simulink library "pmm"  (R2021b)
settings: Solver=VariableStepAuto  StartTime=0.0  StopTime=10.0  RelTol=1e-3
undefined symbols (not defined in the file or in its folder): ENUM_ACMAINRLYSTS_OPEN, ENUM_ACPRECHRGRLYSTS_OPEN, ENUM_B2VRLYSTA_OPEN, ENUM_BMSHVSTS_HVOPEN, ENUM_BRAKEPEDAL_RELEASED, ENUM_CACRLYDEM_CLOSE, ENUM_CACRLYSTS_OPEN, ENUM_CHRGFAULT_ACRLYFAIL, ENUM_CHRGFAULT_BCUHVFAIL, ENUM_CHRGFAULT_BCUNEGFAIL, ENUM_CHRGFAULT_BCUTIMEOUT, ENUM_CHRGFAULT_DCDCENABLE, ENUM_CHRGFAULT_DCDCRLYFAIL, ENUM_CHRGFAULT_HVILFAIL, ENUM_CHRGFAULT_PDUHVFAIL, ENUM_CHRGFAULT_RLYCHKFAIL, ENUM_DCDCEACPCURLYSTA_CLOSED, ENUM_DCDCEACPCURLYSTA_FAILTOCLOSE, ENUM_DCDCEACPCURLYSTA_OPEN, ENUM_DCDCEACPCURLYSTA_WELDED, ENUM_DCDCENABLESTS_READY, ENUM_DCDCRLYSTS_OPEN, ENUM_EHPSRLYDEM_CLOSE, ENUM_EHPSRLYSTS_OPEN, ENUM_FOGRLYENCMD_DISABLE, ENUM_GEARACTUALPOSN_D, ENUM_HVPWROFFREQ_POWEROFF, ENUM_KEYSTATUS_OFF, ENUM_KEYSTATUS_ON, ENUM_KEYSTATUS_START, ENUM_LOWBATTVOLTAGE_NORMAL, ENUM_LOWBATTVOLTAGE_POWERDOWN, ENUM_LOWBATTVOLTAGE_POWERUP, ENUM_MCUHVLOOP_POWEROFF, ENUM_MCUHVLOOPSTS_OPEN, ENUM_MCUMAINRLYSTS_OPEN, ENUM_MCUPRECHRGRLYSTS_OPEN, ENUM_PDFAULT_ACRLYOPEN, ENUM_PDFAULT_BCUDISABLE, ENUM_PDFAULT_DCDCDISABLE, ENUM_PDFAULT_DCDCRLYOPEN, ENUM_PDFAULT_EACDISABLE, ENUM_PDFAULT_EACRLYOPEN, ENUM_PDFAULT_EHPSDISABLE, ENUM_PDFAULT_EHPSRLYOPEN, ENUM_PDFAULT_MCUDISABLE, ENUM_PDFAULT_MCUDISCHRG, ENUM_PDFAULT_MCURLYOPEN, ENUM_PEUSELFCHKSTS_NOFAULT, ENUM_PLUGINSTS_NOPLUGIN, ENUM_PLUGINSTS_PLUGIN, ENUM_PMMMODE_DRIVE, ENUM_PMMMODE_LVBATCHRG, ENUM_PUSTATE_DCDCENABLE, ENUM_PUSTATE_EACPRESCHECK, ENUM_PUSTATE_EHPSENABLE, ENUM_PUSTATE_MCUENABLE, ENUM_PUSTATE_PDUMCURLYCLOSED, ENUM_PUSTATE_POWERUPFAIL, ENUM_TARGETGEAR_REVERSE ... (+126)
libraries: hcu_lib x45, simulink x5, ddm x1, dsc x1
(part 4 of 7)

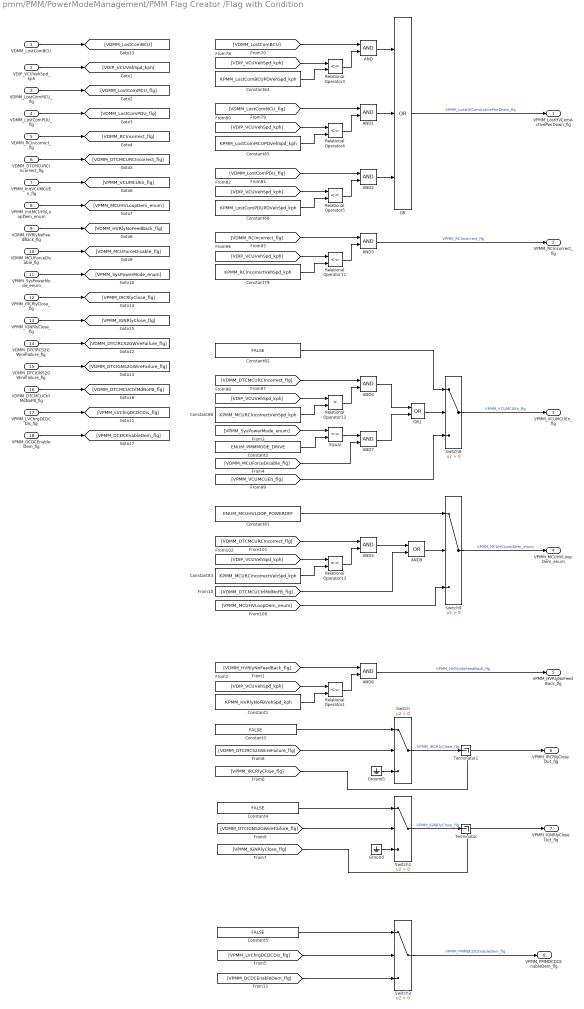
== system pmm/PMM/PowerModeManagement/PMM Flag Creator /Flag with Condition ==
  VDMM_LostComBCU : Inport
  VDIP_VCUVehSpd_kph : Inport  Port=2
  VDMM_LostComMCU_flg : Inport  Port=3
  VDMM_LostComPDU_flg : Inport  Port=4
  VDMM_RCIncorrect_flg : Inport  Port=5
  VDMM_DTCMCURCIncorrect_flg : Inport  Port=6
  VPMM_InitVCUMCUEn_flg : Inport  Port=7
  VPMM_InitMCUHVLoopDem_enum : Inport  Port=8
  VDMM_HVRlyNoFeedBack_flg : Inport  Port=9
  VDMM_MCUForceDisable_flg : Inport  Port=10
  VPMM_SysPowerMode_enum : Inport  Port=11
  VPMM_IRCRlyClose_flg : Inport  Port=12
  VPMM_IGNRlyClose_flg : Inport  Port=13
  VDMM_DTCIRCS2GWireFailure_flg : Inport  Port=14
  VDMM_DTCIGNS2GWireFailure_flg : Inport  Port=15
  VDMM_DTCMCUCtrlMdNoFB_flg : Inport  Port=16
  VPMM_LVChrgDCDCDis_flg : Inport  Port=17
  VPMM_DCDCEnableDem_flg : Inport  Port=18
  AND{,1..7} (8 alike) : Logic  AllPortsSameDT=off  OutDataTypeStr=boolean
  AND9 : Logic  Operator=OR  AllPortsSameDT=off  OutDataTypeStr=boolean
  Constant1 : Constant  Value=KPMM_HVRlyNoFBVehSpd_kph
  Constant2 : Constant  Value=ENUM_PMMMODE_DRIVE
  Constant{3..5,82} (4 alike) : Constant  Value=FALSE
  Constant64 : Constant  Value=KPMM_LostComBCUPDVehSpd_kph
  Constant65 : Constant  Value=KPMM_LostComMCUPDVehSpd_kph
  Constant66 : Constant  Value=KPMM_LostComPDUPDVehSpd_kph
  Constant79 : Constant  Value=KPMM_RCIncorrectVehSpd_kph
  Constant80 : Constant  Value=KPMM_MCURCIncorrectVehSpd_kph
  Constant81 : Constant  Value=ENUM_MCUHVLOOP_POWEROFF
  Constant83 : Constant  Value=KPMM_MCURCIncorrectVehSpd_kph
  Equal : RelationalOperator  Operator===  OutDataTypeStr=boolean  RndMeth=Simplest
  Ground : Ground
  Ground1 : Ground
  OR : Logic  Operator=OR  Inputs=3  AllPortsSameDT=off  OutDataTypeStr=boolean
  OR1 : Logic  Operator=OR  AllPortsSameDT=off  OutDataTypeStr=boolean
  Relational Operator{1,3..5,11,13} (6 alike) : RelationalOperator  Operator=<=  OutDataTypeStr=boolean  RndMeth=Simplest
  Relational Operator12 : RelationalOperator  Operator=>  OutDataTypeStr=boolean  RndMeth=Simplest
  Switch{,1..2,8..9} (5 alike) : Switch  Criteria=u2 > Threshold
  Terminator : Terminator
  Terminator1 : Terminator
  VPMM_LostHVComActivePwrDown_flg : Outport
  VPMM_RCIncorrect_flg : Outport  Port=2
  VPMM_VCUMCUEn_flg : Outport  Port=3
  VPMM_MCUHVLoopDem_enum : Outport  Port=4
  VPMM_HVRlyNoFeedBack_flg : Outport  Port=5
  VPMM_IRCRlyCloseOut_flg : Outport  Port=6
  VPMM_IGNRlyCloseOut_flg : Outport  Port=7
  VPMM_PMMDCDCEnableDem_flg : Outport  Port=8
  wires:
  Relational Operator11/1 -> AND3/2
  Relational Operator4/1 -> AND1/2
  Constant79/1 -> Relational Operator11/2
  AND/1 -> OR/1
  Relational Operator5/1 -> AND2/2
  [VDIP_VCUVehSpd_kph] -> Relational Operator3/1
  [VDIP_VCUVehSpd_kph] -> Relational Operator11/1
  Relational Operator12/1 -> AND4/2
  [VDMM_LostComPDU_flg] -> AND2/1
  [VDMM_DTCMCURCIncorrect_flg] -> AND5/1
  Constant65/1 -> Relational Operator4/2
  Constant83/1 -> Relational Operator13/2
  OR/1 -> VPMM_LostHVComActivePwrDown_flg/1  "VPMM_LostHVComActivePwrDown_flg"
  [VDIP_VCUVehSpd_kph] -> Relational Operator12/1
  Constant80/1 -> Relational Operator12/2
  Relational Operator13/1 -> AND5/2
  Constant66/1 -> Relational Operator5/2
  [VDIP_VCUVehSpd_kph] -> Relational Operator5/1
  [VDMM_LostComBCU] -> AND/1
  Constant64/1 -> Relational Operator3/2
  AND2/1 -> OR/3
  Relational Operator3/1 -> AND/2
  [VDMM_LostComMCU_flg] -> AND1/1
  [VDMM_RCIncorrect_flg] -> AND3/1
  [VDIP_VCUVehSpd_kph] -> Relational Operator4/1
  [VDIP_VCUVehSpd_kph] -> Relational Operator13/1
  AND1/1 -> OR/2
  Switch8/1 -> VPMM_VCUMCUEn_flg/1  "VPMM_VCUMCUEn_flg"
  Switch9/1 -> VPMM_MCUHVLoopDem_enum/1  "VPMM_MCUHVLoopDem_enum"
  AND3/1 -> VPMM_RCIncorrect_flg/1  "VPMM_RCIncorrect_flg"
  VDMM_LostComBCU/1 -> [VDMM_LostComBCU]
  VDIP_VCUVehSpd_kph/1 -> [VDIP_VCUVehSpd_kph]
  VDMM_LostComMCU_flg/1 -> [VDMM_LostComMCU_flg]
  VDMM_LostComPDU_flg/1 -> [VDMM_LostComPDU_flg]
  VDMM_RCIncorrect_flg/1 -> [VDMM_RCIncorrect_flg]
  VDMM_DTCMCURCIncorrect_flg/1 -> [VDMM_DTCMCURCIncorrect_flg]
  VPMM_InitVCUMCUEn_flg/1 -> [VPMM_VCUMCUEn_flg]
  VPMM_InitMCUHVLoopDem_enum/1 -> [VPMM_MCUHVLoopDem_enum]
  AND6/1 -> VPMM_HVRlyNoFeedBack_flg/1  "VPMM_HVRlyNoFeedBack_flg"
  [VDMM_HVRlyNoFeedBack_flg] -> AND6/1
  [VDIP_VCUVehSpd_kph] -> Relational Operator1/1
  Constant1/1 -> Relational Operator1/2
  Relational Operator1/1 -> AND6/2
  VDMM_HVRlyNoFeedBack_flg/1 -> [VDMM_HVRlyNoFeedBack_flg]
  VDMM_MCUForceDisable_flg/1 -> [VDMM_MCUForceDisable_flg]
  VPMM_SysPowerMode_enum/1 -> [VPMM_SysPowerMode_enum]
  [VPMM_SysPowerMode_enum] -> Equal/1
  Constant2/1 -> Equal/2
  Equal/1 -> AND7/1
  [VDMM_MCUForceDisable_flg] -> AND7/2
  OR1/1 -> Switch8/2
  AND4/1 -> OR1/1
  AND7/1 -> OR1/2
  [VPMM_VCUMCUEn_flg] -> Switch8/3
  Constant82/1 -> Switch8/1
  [VDMM_DTCMCURCIncorrect_flg] -> AND4/1
  VDMM_DTCIGNS2GWireFailure_flg/1 -> [VDMM_DTCIGNS2GWireFailure_flg]
  VDMM_DTCIRCS2GWireFailure_flg/1 -> [VDMM_DTCIRCS2GWireFailure_flg]
  VPMM_IGNRlyClose_flg/1 -> [VPMM_IGNRlyClose_flg]
  VPMM_IRCRlyClose_flg/1 -> [VPMM_IRCRlyClose_flg]
  [VDMM_DTCIRCS2GWireFailure_flg] -> Switch/2
  Constant3/1 -> Switch/1
  Constant4/1 -> Switch1/1
  VDMM_DTCMCUCtrlMdNoFB_flg/1 -> [VDMM_DTCMCUCtrlMdNoFB_flg]
  AND5/1 -> AND9/1
  AND9/1 -> Switch9/2
  [VDMM_DTCMCUCtrlMdNoFB_flg] -> AND9/2
  [VPMM_MCUHVLoopDem_enum] -> Switch9/3
  Constant81/1 -> Switch9/1
  [VDMM_DTCIGNS2GWireFailure_flg] -> Switch1/2
  [VPMM_IGNRlyClose_flg] -> VPMM_IGNRlyCloseOut_flg/1
  Switch1/1 -> Terminator/1  "VPMM_IGNRlyClose_flg"
  Ground/1 -> Switch1/3
  [VPMM_IRCRlyClose_flg] -> VPMM_IRCRlyCloseOut_flg/1
  Ground1/1 -> Switch/3
  Switch/1 -> Terminator1/1  "VPMM_IRCRlyClose_flg"
  VPMM_LVChrgDCDCDis_flg/1 -> [VPMM_LVChrgDCDCDis_flg]
  [VPMM_LVChrgDCDCDis_flg] -> Switch2/2
  Constant5/1 -> Switch2/1
  VPMM_DCDCEnableDem_flg/1 -> [VPMM_DCDCEnableDem_flg]
  [VPMM_DCDCEnableDem_flg] -> Switch2/3
  Switch2/1 -> VPMM_PMMDCDCEnableDem_flg/1  "VPMM_PMMDCDCEnableDem_flg"

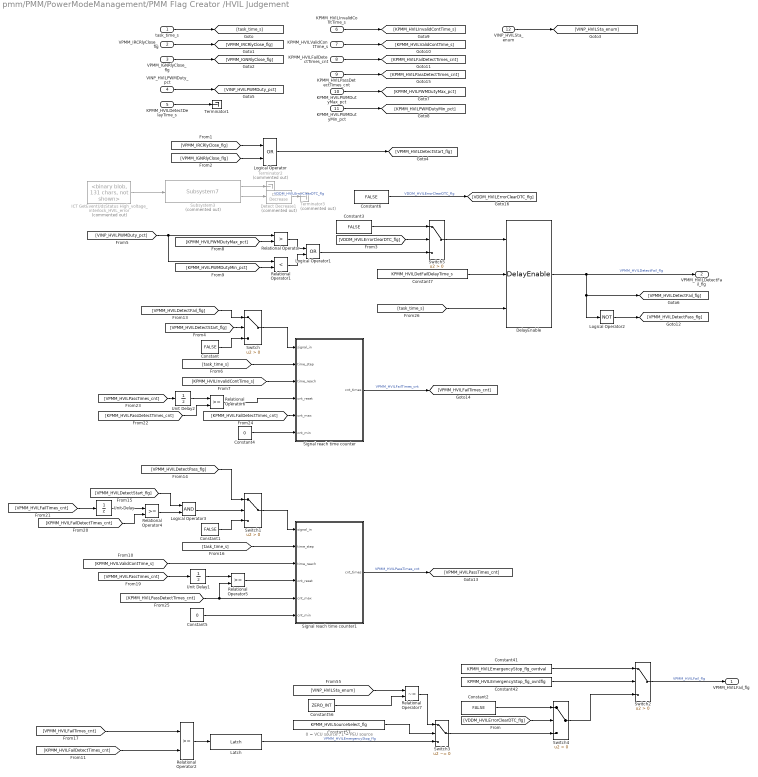
== system pmm/PMM/PowerModeManagement/PMM Flag Creator /HVIL Judgement ==
  note: 0 = VCU source；1 = PEU source
  task_time_s : Inport
  VPMM_IRCRlyClose_flg : Inport  Port=2
  VPMM_IGNRlyClose_flg : Inport  Port=3
  VINP_HVILPWMDuty_pct : Inport  Port=4
  KPMM_HVILDetectDelayTime_s : Inport  Port=5
  KPMM_HVILInvalidContTime_s : Inport  Port=6
  KPMM_HVILValidContTime_s : Inport  Port=7
  KPMM_HVILFailDetectTimes_cnt : Inport  Port=8
  KPMM_HVILPassDetectTimes_cnt : Inport  Port=9
  KPMM_HVILPWMDutyMax_pct : Inport  Port=10
  KPMM_HVILPWMDutyMin_pct : Inport  Port=11
  VINP_HVILSta_enum : Inport  Port=12
  Constant{,1..3,6} (5 alike) : Constant  Value=FALSE
  Constant4 : Constant  Value=0  OutDataTypeStr=single
  Constant41 : Constant  Value=KPMM_HVILEmergencyStop_flg_ovrdval
  Constant42 : Constant  Value=KPMM_HVILEmergencyStop_flg_ovrdflg
  Constant5 : Constant  Value=0  OutDataTypeStr=single
  Constant56 : Constant  Value=ZERO_INT
  Constant57 : Constant  Value=KPMM_HVILSourceSelect_flg
  Constant7 : Constant  Value=KPMM_HVILDetFailDelayTime_s
  DelayEnable : hcu_lib/Basic_Blocks/DelayEnable
  Detect Decrease1 : simulink/Logic and Bit Operations/Detect Decrease  Commented=on  vinit=0.0  OutDataTypeStr=boolean
  ICT GetEventUdsStatus High_voltage_interlock_HVIL_error : ddm/DDM/DMM_Module/SOP3 Wire Failure Detection/Rolling Counting Error Clear/ICT GetEventUdsStatus High_voltage_interlock_HVIL_error  Commented=on  SystemSampleTime=-1  VariantActivationTime=update diagram  Latency=0  AutoFrameSizeCalculation=off
  Latch : hcu_lib/Basic_Blocks/Latch
  Logical Operator : Logic  Operator=OR  AllPortsSameDT=off  OutDataTypeStr=boolean
  Logical Operator1 : Logic  Operator=OR  AllPortsSameDT=off  OutDataTypeStr=boolean
  Logical Operator2 : Logic  Operator=NOT  AllPortsSameDT=off  OutDataTypeStr=boolean
  Logical Operator3 : Logic  AllPortsSameDT=off  OutDataTypeStr=boolean
  Relational Operator : RelationalOperator  Operator=>  OutDataTypeStr=boolean  RndMeth=Simplest
  Relational Operator1 : RelationalOperator  Operator=<  OutDataTypeStr=boolean  RndMeth=Simplest
  Relational Operator{2,4..6} (4 alike) : RelationalOperator  OutDataTypeStr=boolean  RndMeth=Simplest
  Relational Operator7 : RelationalOperator  Operator=~=  OutDataTypeStr=boolean  RndMeth=Simplest
  Signal reach time counter : Subsystem
  Signal reach time counter1 : Subsystem
  Subsystem3 : dsc/DSC/DSC/DTC_DMM/Subsystem7  Commented=on  SystemSampleTime=-1  VariantActivationTime=update diagram  Latency=0  AutoFrameSizeCalculation=off
  Switch{,1..2,4..5} (5 alike) : Switch  Criteria=u2 > Threshold
  Switch3 : Switch  Criteria=u2 ~= 0
      settings: AttributesFormatString=%<Criteria>
  Terminator1 : Terminator
  Terminator2 : Terminator  Commented=on
  Terminator3 : Terminator  Commented=on
  Unit Delay : UnitDelay  SampleTime=-1  HasFrameUpgradeWarning=on
  Unit Delay1 : UnitDelay  SampleTime=-1  HasFrameUpgradeWarning=on
  Unit Delay2 : UnitDelay  SampleTime=-1  HasFrameUpgradeWarning=on
  VPMM_HVILFail_flg : Outport
  VPMM_HVILDetectFail_flg : Outport  Port=2
  wires:
  Logical Operator1/1 -> Switch5/3
  [VDDM_HVILErrorClearDTC_flg] -> Switch5/2
  Constant3/1 -> Switch5/1
  Switch4/1 -> Switch2/3
  Constant2/1 -> Switch4/1
  [VDDM_HVILErrorClearDTC_flg] -> Switch4/2
  Switch3/1 -> Switch4/3
  Constant6/1 -> [VDDM_HVILErrorClearDTC_flg]  "VDDM_HVILErrorClearDTC_flg"
  Subsystem3/2 -> Detect Decrease1/1
  ICT GetEventUdsStatus High_voltage_interlock_HVIL_error/1 -> Subsystem3/1
  Subsystem3/1 -> Terminator2/1
  Unit Delay2/1 -> Relational Operator6/1
  Unit Delay1/1 -> Relational Operator5/1
  Unit Delay/1 -> Relational Operator4/1
  [VPMM_HVILPassTimes_cnt] -> Unit Delay2/1
  [KPMM_HVILPassDetectTimes_cnt] -> Relational Operator6/2
  Relational Operator6/1 -> Signal reach time counter/4(cnt_reset)
  [VPMM_HVILPassTimes_cnt] -> Unit Delay1/1
  Logical Operator3/1 -> Switch1/2
  [VPMM_HVILDetectStart_flg] -> Logical Operator3/1
  [KPMM_HVILFailDetectTimes_cnt] -> Relational Operator4/2
  Relational Operator4/1 -> Logical Operator3/2
  [VPMM_HVILFailTimes_cnt] -> Unit Delay/1
  Relational Operator5/1 -> Signal reach time counter1/4(cnt_reset)
  Relational Operator2/1 -> Latch/1
  [KPMM_HVILFailDetectTimes_cnt] -> Relational Operator2/2
  [VPMM_HVILFailTimes_cnt] -> Relational Operator2/1
  KPMM_HVILPassDetectTimes_cnt/1 -> [KPMM_HVILPassDetectTimes_cnt]
  [KPMM_HVILValidContTime_s] -> Signal reach time counter1/3(time_reach)
  [task_time_s] -> Signal reach time counter1/2(time_step)
  [VPMM_HVILDetectPass_flg] -> Switch1/1
  Switch1/1 -> Signal reach time counter1/1(signal_in)
  Constant1/1 -> Switch1/3
  [KPMM_HVILPassDetectTimes_cnt] -> Signal reach time counter1/5(cnt_max), Relational Operator5/2
  Constant5/1 -> Signal reach time counter1/6(cnt_min)
  Signal reach time counter1/1(cnt_times) -> [VPMM_HVILPassTimes_cnt]  "VPMM_HVILPassTimes_cnt"
  Signal reach time counter/1(cnt_times) -> [VPMM_HVILFailTimes_cnt]  "VPMM_HVILFailTimes_cnt"
  Constant4/1 -> Signal reach time counter/6(cnt_min)
  [KPMM_HVILFailDetectTimes_cnt] -> Signal reach time counter/5(cnt_max)
  Constant/1 -> Switch/3
  [VPMM_HVILDetectStart_flg] -> Switch/2
  Switch/1 -> Signal reach time counter/1(signal_in)
  [VPMM_HVILDetectFail_flg] -> Switch/1
  [task_time_s] -> Signal reach time counter/2(time_step)
  [KPMM_HVILInvalidContTime_s] -> Signal reach time counter/3(time_reach)
  Logical Operator2/1 -> [VPMM_HVILDetectPass_flg]
  Relational Operator1/1 -> Logical Operator1/2
  Relational Operator/1 -> Logical Operator1/1
  [KPMM_HVILPWMDutyMin_pct] -> Relational Operator1/2
  [KPMM_HVILPWMDutyMax_pct] -> Relational Operator/2
  [VINP_HVILPWMDuty_pct] -> Relational Operator/1, Relational Operator1/1
  KPMM_HVILFailDetectTimes_cnt/1 -> [KPMM_HVILFailDetectTimes_cnt]
  KPMM_HVILValidContTime_s/1 -> [KPMM_HVILValidContTime_s]
  KPMM_HVILInvalidContTime_s/1 -> [KPMM_HVILInvalidContTime_s]
  KPMM_HVILPWMDutyMin_pct/1 -> [KPMM_HVILPWMDutyMin_pct]
  KPMM_HVILPWMDutyMax_pct/1 -> [KPMM_HVILPWMDutyMax_pct]
  VINP_HVILPWMDuty_pct/1 -> [VINP_HVILPWMDuty_pct]
  Logical Operator/1 -> [VPMM_HVILDetectStart_flg]
  KPMM_HVILDetectDelayTime_s/1 -> Terminator1/1
  [VPMM_IGNRlyClose_flg] -> Logical Operator/2
  [VPMM_IRCRlyClose_flg] -> Logical Operator/1
  VPMM_IGNRlyClose_flg/1 -> [VPMM_IGNRlyClose_flg]
  VPMM_IRCRlyClose_flg/1 -> [VPMM_IRCRlyClose_flg]
  task_time_s/1 -> [task_time_s]
  Relational Operator7/1 -> Switch3/1
  [VINP_HVILSta_enum] -> Relational Operator7/1
  Switch2/1 -> VPMM_HVILFail_flg/1  "VPMM_HVILFail_flg"
  Constant57/1 -> Switch3/2
  Constant56/1 -> Relational Operator7/2
  Constant41/1 -> Switch2/1
  Latch/1 -> Switch3/3  "VPMM_HVILEmergencyStop_flg"
  Constant42/1 -> Switch2/2
  VINP_HVILSta_enum/1 -> [VINP_HVILSta_enum]
  Detect Decrease1/1 -> Terminator3/1  "VDDM_HVILErrorClearDTC_flg"
  Switch5/1 -> DelayEnable/1
  DelayEnable/1 -> Logical Operator2/1, [VPMM_HVILDetectFail_flg], VPMM_HVILDetectFail_flg/1  "VPMM_HVILDetectFail_flg"
  [task_time_s] -> DelayEnable/3
  Constant7/1 -> DelayEnable/2

== system pmm/PMM/PowerModeManagement/PMM Flag Creator /Long Idle Detection ==
  VDIP_VCUVehSpd_kph : Inport
  VTQD_GearActualPosn_enum : Inport  Port=2
  VINP_EBSBrakeSw_enum : Inport  Port=3
  VINP_MotorSpd_rpm : Inport  Port=4
  VSCP_FRDoorOPSta_flg : Inport  Port=5
  VSCP_MDDoorOPSta_flg : Inport  Port=6
  VSCP_TDDoorOPSta_flg : Inport  Port=7
  VPMM_SysPowerMode_enum : Inport  Port=8
  task_time_s : Inport  Port=9
  AND : Logic  Inputs=4  AllPortsSameDT=off  OutDataTypeStr=boolean
  AND1 : Logic  Inputs=3  AllPortsSameDT=off  OutDataTypeStr=boolean
  AND2 : Logic  AllPortsSameDT=off  OutDataTypeStr=boolean
  Abs : Abs
  Constant : Constant  Value=KPMM_LongIdleDectVehSpd_kph
  Constant1 : Constant  Value=ENUM_GEARACTUALPOSN_D
  Constant2 : Constant  Value=KPMM_LongIdleDectMotorSpd_rpm
  Constant3 : Constant  Value=ENUM_PMMMODE_DRIVE
  Constant4 : Constant  Value=KPMM_LongIdleDectTime_s
  Constant5 : Constant  Value=KPMM_LongIdleDetSW_flg
  Constant6 : Constant  Value=ENUM_BRAKEPEDAL_RELEASED
  Constant7 : Constant  Value=KPMM_LongIdleBuzzerFlashTime_s
  DelayEnable : hcu_lib/Basic_Blocks/DelayEnable
  DelayEnable1 : hcu_lib/Basic_Blocks/DelayEnable
  Equal : RelationalOperator  Operator===  OutDataTypeStr=boolean  RndMeth=Simplest
  Equal1 : RelationalOperator  Operator===  OutDataTypeStr=boolean  RndMeth=Simplest
  Equal2 : RelationalOperator  Operator===  OutDataTypeStr=boolean  RndMeth=Simplest
  Latch : hcu_lib/Basic_Blocks/Latch
  OR : Logic  Operator=OR  Inputs=3  AllPortsSameDT=off  OutDataTypeStr=boolean
  Relational Operator : RelationalOperator  Operator=<=  OutDataTypeStr=boolean  RndMeth=Simplest
  Relational Operator1 : RelationalOperator  Operator=<=  OutDataTypeStr=boolean  RndMeth=Simplest
  VPMM_LongIdleDetFinsh_flg : Outport
  VPMM_LongIdle_flg : Outport  Port=2
  wires:
  AND1/1 -> DelayEnable/1  "VPMM_LongIdleEn_flg"
  task_time_s/1 -> [task_time_s]
  [VDIP_VCUVehSpd_kph] -> Relational Operator/1
  [VPMM_LongIdleDoorCon_flg] -> AND1/2
  DelayEnable/1 -> Latch/1
  Latch/1 -> AND2/1
  Constant5/1 -> AND2/2
  Equal/1 -> AND/2
  Constant4/1 -> DelayEnable/2
  AND2/1 -> [VPMM_LongIdleDetFinsh_flg]  "VPMM_LongIdleDetFinsh_flg"
  OR/1 -> [VPMM_LongIdleDoorCon_flg]  "VPMM_LongIdleDoorCon_flg"
  VINP_EBSBrakeSw_enum/1 -> [VINP_EBSBrakeSw_enum]
  [VPMM_LongIdleDetFinsh_flg] -> VPMM_LongIdleDetFinsh_flg/1
  VDIP_VCUVehSpd_kph/1 -> [VDIP_VCUVehSpd_kph]
  Constant1/1 -> Equal/2
  Constant/1 -> Relational Operator/2
  Constant2/1 -> Relational Operator1/2
  VSCP_FRDoorOPSta_flg/1 -> [VSCP_FRDoorOPSta_flg]
  [VPMM_SysPowerMode_enum] -> Equal1/1
  VINP_MotorSpd_rpm/1 -> [VINP_MotorSpd_rpm]
  Abs/1 -> Relational Operator1/1
  Relational Operator1/1 -> AND/3
  Equal2/1 -> AND/4
  [VPMM_LongIdlePowerCon_flg] -> AND1/3
  Relational Operator/1 -> AND/1
  VSCP_MDDoorOPSta_flg/1 -> [VSCP_MDDoorOPSta_flg]
  Equal1/1 -> [VPMM_LongIdlePowerCon_flg]  "VPMM_LongIdlePowerCon_flg"
  AND/1 -> [VPMM_LongIdleDriveCon_flg]  "VPMM_LongIdleDriveCon_flg"
  VTQD_GearActualPosn_enum/1 -> [VTQD_GearActualPosn_enum]
  [VPMM_LongIdleDriveCon_flg] -> AND1/1
  VSCP_TDDoorOPSta_flg/1 -> [VSCP_TDDoorOPSta_flg]
  [task_time_s] -> DelayEnable/3
  VPMM_SysPowerMode_enum/1 -> [VPMM_SysPowerMode_enum]
  Constant3/1 -> Equal1/2
  Constant6/1 -> Equal2/2
  [VINP_MotorSpd_rpm] -> Abs/1
  [VINP_EBSBrakeSw_enum] -> Equal2/1
  [VTQD_GearActualPosn_enum] -> Equal/1
  [VPMM_LongIdleDetFinsh_flg] -> DelayEnable1/1
  Constant7/1 -> DelayEnable1/2
  [task_time_s] -> DelayEnable1/3
  DelayEnable1/1 -> [VPMM_LongIdle_flg]  "VPMM_LongIdle_flg"
  [VPMM_LongIdle_flg] -> VPMM_LongIdle_flg/1
  [VSCP_FRDoorOPSta_flg] -> OR/1
  [VSCP_MDDoorOPSta_flg] -> OR/2
  [VSCP_TDDoorOPSta_flg] -> OR/3

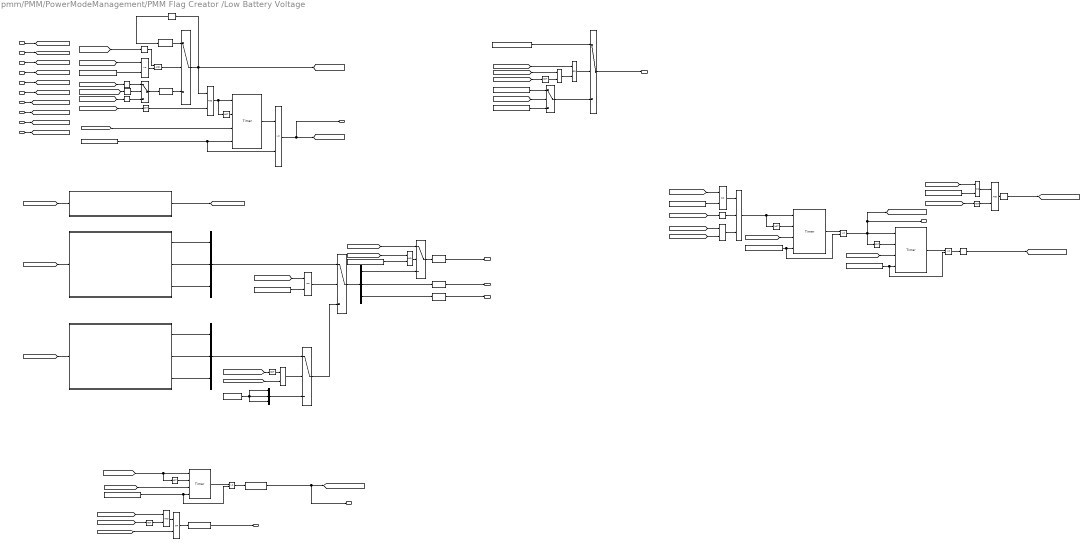
== system pmm/PMM/PowerModeManagement/PMM Flag Creator /Low Battery Voltage ==
  note: LVChrgMode Cycle Timer
  note: Battery Low Voltage Indicator
  note: Flasher
  note: Low Valtage Detection
  task_time_s : Inport
  VINP_DCDCOutVol_V : Inport  Port=2
  VINP_DCDCEnSta_enum : Inport  Port=3
  VPMM_LVChrgIinit2Idle_flg : Inport  Port=4
  VPMM_SysPowerMode_enum : Inport  Port=5
  VINP_B2VSOC_pct : Inport  Port=6
  VPMM_HVUnitSelfChkCompleted4PU_flg : Inport  Port=7
  VPMM_LVChrgInit2PowerUp_flg : Inport  Port=8
  VPMM_HVILFail_flg : Inport  Port=9
  VPMM_LongIdleDetFinsh_flg : Inport  Port=10
  AND{,1,4..8} (7 alike) : Logic  AllPortsSameDT=off  OutDataTypeStr=boolean
  AND2 : Logic  Inputs=3  AllPortsSameDT=off  OutDataTypeStr=boolean
  AND3 : Logic  Operator=NAND  AllPortsSameDT=off  OutDataTypeStr=boolean
  Constant1 : Constant  Value=ENUM_LOWBATTVOLTAGE_NORMAL  VectorParams1D=off
  Constant10 : Constant  Value=KPMM_LongIdleBuzzerSW_flg  VectorParams1D=off
  Constant2 : Constant  Value=ENUM_LOWBATTVOLTAGE_POWERUP  VectorParams1D=off
  Constant20 : Constant  Value=FALSE
  Constant3 : Constant  Value=KPMM_LVChrgPreAction_s  VectorParams1D=off
  Constant4 : Constant  Value=ENUM_LOWBATTVOLTAGE_POWERDOWN  VectorParams1D=off
  Constant5 : Constant  Value=ENUM_PMMMODE_LVBATCHRG  VectorParams1D=off
  Constant6 : Constant  Value=ENUM_PMMMODE_LVBATCHRG  VectorParams1D=off
  Constant7 : Constant  Value=KPMM_LVChrgDCDCEnTimer_s  VectorParams1D=off
  Constant76 : Constant  Value=KPMM_LVChrgPreAlarm_s  VectorParams1D=off
  Constant78 : Constant  Value=ENUM_DCDCENABLESTS_READY
  Constant8 : Constant  Value=KPMM_LVChrgDCDCDisTimer_s  VectorParams1D=off
  Constant9 : Constant  Value=ENUM_PMMMODE_LVBATCHRG  VectorParams1D=off
  Data Type Conversion{,1..4} (5 alike) : DataTypeConversion  OutDataTypeStr=boolean
  Delay{,1..4} (5 alike) : Delay  DelayLength=1
  Demux : Demux  Outputs=3
  Equal : RelationalOperator  Operator===  OutDataTypeStr=boolean  RndMeth=Simplest
  Equal1 : RelationalOperator  Operator===  OutDataTypeStr=boolean  RndMeth=Simplest
  Equal2 : RelationalOperator  Operator===  OutDataTypeStr=boolean  RndMeth=Simplest
  Latch : hcu_lib/Basic_Blocks/Latch
  Latch1 : hcu_lib/Basic_Blocks/Latch
  Long Idle Flasher : Subsystem
  Low Voltage Charge Action Flasher : Subsystem
  Low Voltage Charge Pre-Action Flasher : Subsystem
  Mux : Mux  Inputs=3
  Mux1 : Mux  Inputs=3
  Mux2 : Mux  Inputs=3
  NOT{,1..8} (9 alike) : Logic  Operator=NOT  AllPortsSameDT=off  OutDataTypeStr=boolean
  OR : Logic  Operator=OR  AllPortsSameDT=off  OutDataTypeStr=boolean
  OR2 : Logic  Operator=OR  AllPortsSameDT=off  OutDataTypeStr=boolean
  Relational Operator{,1..2,9} (4 alike) : RelationalOperator  OutDataTypeStr=boolean  RndMeth=Simplest
  Relational Operator10 : RelationalOperator  Operator=~=  OutDataTypeStr=boolean  RndMeth=Simplest
  Relay : Relay  OnSwitchValue=KPMM_LVChrgDisVoltageDet_V  OffSwitchValue=KPMM_LVChrgEnVoltageDet_V  OnOutputValue=FALSE  OffOutputValue=TRUE
  Relay1 : Relay  OnSwitchValue=KPMM_LVChrgDisVoltageDur_V  OffSwitchValue=KPMM_LVChrgEnVoltageDur_V  OnOutputValue=FALSE  OffOutputValue=TRUE
  Relay2 : Relay  OnSwitchValue=KPMM_LVChrgEnHVSOC_pct  OffSwitchValue=KPMM_LVChrgDisHVSOC_pct  OnOutputValue=TRUE  OffOutputValue=FALSE  OutDataTypeStr=boolean
  Switch{,1..5,7} (7 alike) : Switch  Criteria=u2 > Threshold
  Timer{,1..3} (4 alike) : hcu_lib/Basic_Blocks/Timer
  VPMM_LVBattLowInd_enum : Outport
  VPMM_LVChrgPreActFinished_flg : Outport  Port=2
  VPMM_TrigRBuzeer_flg : Outport  Port=3
  VPMM_TrigRLamp_flg : Outport  Port=4
  VPMM_TrigBrkLamp_flg : Outport  Port=5
  VPMM_LVChrgDCDCDis_flg : Outport  Port=6
  VPMM_LVChrgFinished_flg : Outport  Port=7
  VPMM_DCDCVolLowTO_flg : Outport  Port=8
  wires:
  Timer1/1 -> Relational Operator9/1
  NOT1/1 -> Timer1/2
  Constant78/1 -> Relational Operator10/2
  [VINP_DCDCEnSta_enum] -> Relational Operator10/1
  [task_time_s] -> Timer1/3
  Constant76/1 -> Relational Operator9/2, Timer1/4
  task_time_s/1 -> [task_time_s]
  VINP_DCDCOutVol_V/1 -> [VINP_DCDCOutVol_V]
  VINP_DCDCEnSta_enum/1 -> [VINP_DCDCEnSta_enum]
  Constant1/1 -> Switch/3
  [VINP_DCDCOutVol_V] -> Relay/1
  Constant2/1 -> Switch/1
  [task_time_s] -> Low Voltage Charge Pre-Action Flasher/1(task_time_s)
  Switch7/1 -> Delay/1, [VPMM_LVBattDetLow_flg], AND6/1  "VPMM_LVBattDetLow_flg"
  [VPMM_LVBattDetLow_flg] -> Switch/2
  Relational Operator9/1 -> VPMM_DCDCVolLowTO_flg/1, [VPMM_DCDCVolLowTO_flg]  "VPMM_DCDCVolLowTO_flg"
  NOT/1 -> Timer/2
  [task_time_s] -> Timer/3
  Constant3/1 -> Relational Operator/2, Timer/4
  Timer/1 -> Relational Operator/1
  Low Voltage Charge Pre-Action Flasher/1(VPMM_LVChrgPreActRBuzzer_flg) -> Mux/1
  Low Voltage Charge Pre-Action Flasher/2(VPMM_LVChrgPreActRLamp_flg) -> Mux/2
  Low Voltage Charge Pre-Action Flasher/3(VPMM_LVChrgPreActBrkLamp_flg) -> Mux/3
  AND/1 -> Switch1/2
  Mux/1 -> Switch1/1
  [VPMM_DCDCVolLowTO_flg] -> AND/2
  Mux1/1 -> Switch1/3
  Constant20/1 -> Mux1/3, Mux1/1, Mux1/2
  Switch/1 -> Switch2/3
  Switch2/1 -> VPMM_LVBattLowInd_enum/1  "VPMM_LVBattLowInd_enum"
  Constant4/1 -> Switch2/1
  VPMM_LVChrgIinit2Idle_flg/1 -> [VPMM_LVChrgIinit2Idle_flg]
  Delay/1 -> Data Type Conversion3/1
  NOT2/1 -> AND/1
  [VPMM_LVChrgPreActFinished_flg] -> NOT2/1
  Low Voltage Charge Action Flasher/2(VPMM_LVChrgDuRLamp_flg) -> Mux2/2
  Low Voltage Charge Action Flasher/1(VPMM_LVChrgDuRBuzzer_flg) -> Mux2/1
  Low Voltage Charge Action Flasher/3(VPMM_LVChrgDuBrkLamp_flg) -> Mux2/3
  [task_time_s] -> Low Voltage Charge Action Flasher/1(task_time_s)
  Mux2/1 -> Switch3/1
  Switch1/1 -> Switch3/3
  VPMM_SysPowerMode_enum/1 -> [VPMM_SysPowerMode_enum]
  Equal/1 -> Switch3/2
  [VPMM_SysPowerMode_enum] -> Equal/1
  Constant5/1 -> Equal/2
  Switch3/1 -> Demux/1
  Data Type Conversion/1 -> VPMM_TrigRBuzeer_flg/1  "VPMM_TrigRBuzeer_flg"
  Demux/2 -> Data Type Conversion1/1
  Data Type Conversion1/1 -> VPMM_TrigRLamp_flg/1  "VPMM_TrigRLamp_flg"
  Demux/3 -> Data Type Conversion2/1
  Data Type Conversion2/1 -> VPMM_TrigBrkLamp_flg/1  "VPMM_TrigBrkLamp_flg"
  VINP_B2VSOC_pct/1 -> [VINP_B2VSOC_pct]
  VPMM_HVUnitSelfChkCompleted4PU_flg/1 -> [VPMM_HVUnitSelfChkCompleted4PU_flg]
  NOT4/1 -> AND1/2
  [VPMM_HVUnitSelfChkCompleted4PU_flg] -> NOT4/1
  OR/1 -> Switch2/2
  Constant6/1 -> Equal1/2
  [VPMM_SysPowerMode_enum] -> Equal1/1
  [VINP_B2VSOC_pct] -> Relay2/1
  Equal1/1 -> AND2/1
  Relay2/1 -> AND2/2
  AND2/1 -> NOT6/1, Timer2/1  "VPMM_LVChrgDCDCEn_flg"
  Constant7/1 -> Relational Operator1/2, Timer2/4
  [task_time_s] -> Timer2/3
  Timer2/1 -> Relational Operator1/1
  Relational Operator1/1 -> [VPMM_LVChrgDCDCDis_flg], VPMM_LVChrgDCDCDis_flg/1, NOT5/1, Timer3/1  "VPMM_LVChrgDCDCDis_flg"
  Constant8/1 -> Relational Operator2/2, Timer3/4
  [task_time_s] -> Timer3/3
  NOT5/1 -> Timer3/2
  Timer3/1 -> Relational Operator2/1
  [VPMM_LVChrgDetFinished_flg] -> AND3/1
  [VPMM_LVBattDetLow_flg] -> AND3/2
  NOT6/1 -> Timer2/2
  AND3/1 -> AND2/3
  [VPMM_LVChrgDetFinished_flg] -> AND4/1
  NOT7/1 -> AND4/2
  Relational Operator2/1 -> Delay1/1
  [VPMM_LVChrgPreActFinished_flg] -> AND1/1
  AND1/1 -> OR/2
  [VPMM_LVChrgIinit2Idle_flg] -> OR/1
  Latch/1 -> VPMM_LVChrgFinished_flg/1  "VPMM_LVChrgFinished_flg"
  [VPMM_SysPowerMode_enum] -> Equal2/1
  Constant9/1 -> Equal2/2
  VPMM_LVChrgInit2PowerUp_flg/1 -> [VPMM_LVChrgInit2PowerUp_flg]
  [VPMM_LVChrgInit2PowerUp_flg] -> NOT3/1
  Equal2/1 -> AND5/1
  NOT3/1 -> AND5/2
  Delay1/1 -> [VPMM_LVChrgDetFinished_flg]  "VPMM_LVChrgBattdetEnd_flg"
  AND5/1 -> Delay2/1
  Delay2/1 -> [VPMM_LVChrgDetFault_flg]  "VPMM_LVChrgDetFault_flg"
  AND4/1 -> OR2/1
  OR2/1 -> Latch/1
  [VPMM_LVChrgDetFault_flg] -> OR2/2
  [VPMM_DCDCVolLowTO_flg] -> Timer/1, NOT/1
  [VPMM_LVBattDetLow_flg] -> NOT7/1
  Relay/1 -> Switch4/3
  [VINP_DCDCOutVol_V] -> Relay1/1
  Relay1/1 -> Switch4/1
  Switch4/1 -> Data Type Conversion4/1
  Delay3/1 -> Switch4/2
  [VPMM_LVChrgDCDCDis_flg] -> Delay3/1
  Latch1/1 -> VPMM_LVChrgPreActFinished_flg/1, [VPMM_LVChrgPreActFinished_flg]  "VPMM_LVChrgPreActFinished_flg"
  Relational Operator/1 -> Latch1/1
  AND6/1 -> NOT1/1, Timer1/1
  VPMM_HVILFail_flg/1 -> [VPMM_HVILFail_flg]
  NOT8/1 -> AND6/2
  [VPMM_HVILFail_flg] -> NOT8/1
  Relational Operator10/1 -> AND7/2
  AND7/1 -> Switch7/2
  Delay4/1 -> AND7/1
  [VPMM_DCDCVolLowTO_flg] -> Delay4/1
  [task_time_s] -> Long Idle Flasher/1(task_time_s1)
  Long Idle Flasher/1(VPMM_LongIdleBuzzer_flg) -> [VPMM_LongIdleBuzzer_flg]
  VPMM_LongIdleDetFinsh_flg/1 -> [VPMM_LongIdleDetFinsh_flg]
  Demux/1 -> Switch5/3
  Switch5/1 -> Data Type Conversion/1
  [VPMM_LongIdleBuzzer_flg] -> Switch5/1
  AND8/1 -> Switch5/2
  [VPMM_LongIdleDetFinsh_flg] -> AND8/1
  Constant10/1 -> AND8/2
  Data Type Conversion3/1 -> Switch7/1
  Data Type Conversion4/1 -> Switch7/3

== system pmm/PMM/PowerModeManagement/PMM Flag Creator /MCU Discharge Enable Feedback ==
  task_time_s : Inport
  VINP_AtvDisChgEnFbk_flg : Inport  Port=2
  Constant73 : Constant  Value=KPMM_MCUDisChrgFailtime_s
  Constant74 : Constant  Value=KPMM_MCUDisChrgFailtime_s
  Detect Increase2 : simulink/Logic and Bit Operations/Detect Increase  vinit=0.0  OutDataTypeStr=boolean
  Relational Operator7 : RelationalOperator  OutDataTypeStr=boolean  RndMeth=Simplest
  SR_Latch2 : hcu_lib/Basic_Blocks/SR_Latch
      settings: SourceProductName=HCU Relative Block Library
  Timer : hcu_lib/Basic_Blocks/Timer
      settings: SourceProductName=HCU Relative Block Library
  Unit Delay13 : UnitDelay  SampleTime=-1  HasFrameUpgradeWarning=on
  Unit Delay14 : UnitDelay  SampleTime=-1  HasFrameUpgradeWarning=on
  VPMM_AtvDisChgEnFbk_flg : Outport
  wires:
  Constant74/1 -> Timer/4
  Unit Delay13/1 -> Timer/1
  Detect Increase2/1 -> SR_Latch2/1
  Constant73/1 -> Relational Operator7/2
  Timer/1 -> Relational Operator7/1
  SR_Latch2/1 -> VPMM_AtvDisChgEnFbk_flg/1, Unit Delay13/1  "VPMM_AtvDisChgEnFbk_flg"
  [task_time_s] -> Timer/3
  [VINP_AtvDisChgEnFbk_flg] -> Detect Increase2/1
  Relational Operator7/1 -> SR_Latch2/2, Unit Delay14/1
  Unit Delay14/1 -> Timer/2
  VINP_AtvDisChgEnFbk_flg/1 -> [VINP_AtvDisChgEnFbk_flg]
  task_time_s/1 -> [task_time_s]

== system pmm/PMM/PowerModeManagement/PMM Flag Creator /MCU Status2 Lost Communication ==
  task_time_s : Inport
  VDMM_LostComMCUSta2_flg : Inport  Port=2
  Constant67 : Constant  Value=KPMM_MCUSta2Lost4Sleep_s
  Constant68 : Constant  Value=KPMM_MCUSta2Lost4Sleep_s
  Counter : hcu_lib/Basic_Blocks/Counter
      settings: SourceProductName=HCU Relative Block Library
  Divide1 : Product  Inputs=*/
  NOT : Logic  Operator=NOT  AllPortsSameDT=off  OutDataTypeStr=boolean
  Product : Product
  Relational Operator6 : RelationalOperator  OutDataTypeStr=boolean  RndMeth=Simplest
  VPMM_MCUSta2Lost_flg : Outport
  wires:
  Product/1 -> Relational Operator6/1
  Divide1/1 -> Counter/3
  Counter/1 -> Product/1
  [task_time_s] -> Divide1/2
  [VDMM_LostComMCUSta2_flg] -> Counter/1, NOT/1
  Constant68/1 -> Relational Operator6/2
  [task_time_s] -> Product/2
  Constant67/1 -> Divide1/1
  NOT/1 -> Counter/2
  Relational Operator6/1 -> VPMM_MCUSta2Lost_flg/1  "VPMM_MCUSta2Lost_flg"
  task_time_s/1 -> [task_time_s]
  VDMM_LostComMCUSta2_flg/1 -> [VDMM_LostComMCUSta2_flg]

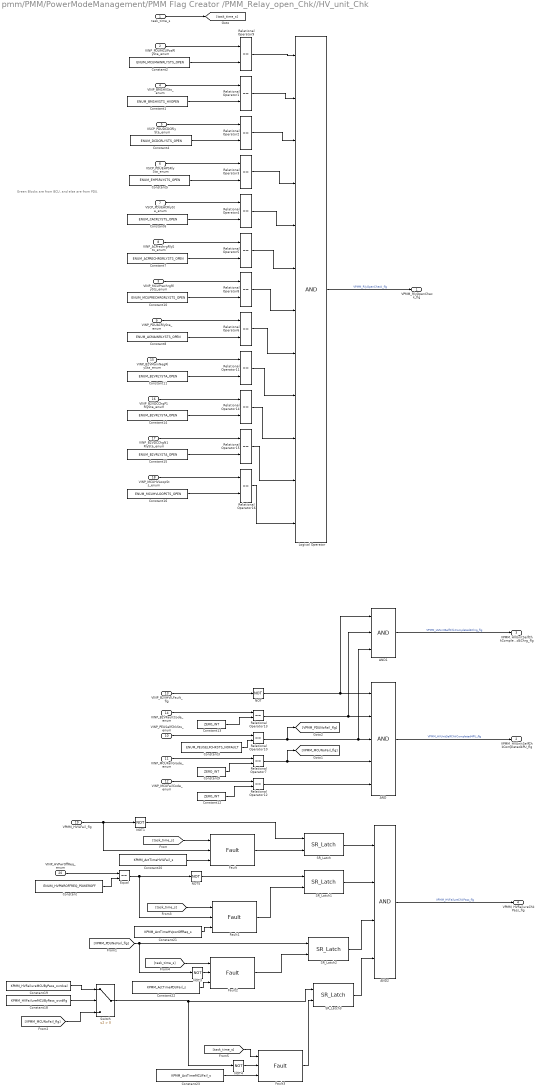
== system pmm/PMM/PowerModeManagement/PMM Flag Creator /PMM_Relay_open_Chk//HV_unit_Chk ==
  note: Green Blocks are from BCU, and else are from PDU.
  task_time_s : Inport
  VINP_PDUMCUPosRlySta_enum : Inport  Port=2
  VINP_MCUPrechrgRlySts_enum : Inport  Port=3
  VINP_BMSHVSts_enum : Inport  Port=4
  VSCP_PDUDCDCRlySta_enum : Inport  Port=5
  VSCP_PDUEHPSRlySta_enum : Inport  Port=6
  VSCP_PDUEACRlySta_enum : Inport  Port=7
  VINP_ACPrechrgRlySts_enum : Inport  Port=8
  VINP_PDUACRlySta_enum : Inport  Port=9
  VINP_PEUSelfChkSts_enum : Inport  Port=10
  VINP_MCUFailGrade_enum : Inport  Port=11
  VINP_MCUFailCode_enum : Inport  Port=12
  VINP_B2VHVILFault_flg : Inport  Port=13
  VINP_B2VFaultCode_enum : Inport  Port=14
  VINP_B2VMainNegRlySta_enum : Inport  Port=15
  VINP_B2VDCChgP1RlySta_enum : Inport  Port=16
  VINP_B2VDCChgN1RlySta_enum : Inport  Port=17
  VINP_MCUHVLoopSts_enum : Inport  Port=18
  VPMM_HVILFail_flg : Inport  Port=19
  VINP_HVPwrOffReq_enum : Inport  Port=20
  AND : Logic  Inputs=5  AllPortsSameDT=off  OutDataTypeStr=boolean
  AND1 : Logic  Inputs=3  AllPortsSameDT=off  OutDataTypeStr=boolean
  AND2 : Logic  Inputs=4  AllPortsSameDT=off  OutDataTypeStr=boolean
  Constant : Constant  Value=ENUM_HVPWROFFREQ_POWEROFF
  Constant1 : Constant  Value=ENUM_BMSHVSTS_HVOPEN
  Constant10 : Constant  Value=ENUM_MCUPRECHRGRLYSTS_OPEN
  Constant11 : Constant  Value=ENUM_B2VRLYSTA_OPEN
  Constant12 : Constant  Value=ZERO_INT
  Constant13 : Constant  Value=ZERO_INT
  Constant14 : Constant  Value=ENUM_B2VRLYSTA_OPEN
  Constant15 : Constant  Value=ENUM_B2VRLYSTA_OPEN
  Constant16 : Constant  Value=ENUM_MCUHVLOOPSTS_OPEN
  Constant18 : Constant  Value=KPMM_HVFailureMCUByPass_ovrdflg
  Constant19 : Constant  Value=KPMM_HVFailureMCUByPass_ovrdval
  Constant2 : Constant  Value=ENUM_MCUMAINRLYSTS_OPEN
  Constant20 : Constant  Value=KPMM_ActTimeHVILFail_s
  Constant21 : Constant  Value=KPMM_ActTimeHVpwrOffReq_s
  Constant22 : Constant  Value=KPMM_ActTimePDUFail_s
  Constant23 : Constant  Value=KPMM_ActTimeMCUFail_s
  Constant3 : Constant  Value=ENUM_PEUSELFCHKSTS_NOFAULT
  Constant4 : Constant  Value=ENUM_DCDCRLYSTS_OPEN
  Constant5 : Constant  Value=ENUM_EHPSRLYSTS_OPEN
  Constant6 : Constant  Value=ENUM_CACRLYSTS_OPEN
  Constant7 : Constant  Value=ENUM_ACPRECHRGRLYSTS_OPEN
  Constant8 : Constant  Value=ENUM_ACMAINRLYSTS_OPEN
  Constant9 : Constant  Value=ZERO_INT
  Equal : RelationalOperator  Operator===  OutDataTypeStr=boolean  RndMeth=Simplest
  Fault{,1..3} (4 alike) : hcu_lib/Basic_Blocks/Fault  SystemSampleTime=-1  VariantActivationTime=update diagram  Latency=0  AutoFrameSizeCalculation=off
      settings: SourceProductName=HCU Relative Block Library
  Logical Operator : Logic  Inputs=12  AllPortsSameDT=off  OutDataTypeStr=boolean
  NOT{,1,3..5} (5 alike) : Logic  Operator=NOT  AllPortsSameDT=off  OutDataTypeStr=boolean
  Relational Operator{1..16} (16 alike) : RelationalOperator  Operator===  OutDataTypeStr=boolean  RndMeth=Simplest
  SR_Latch{,1..3} (4 alike) : hcu_lib/Basic_Blocks/SR_Latch
      settings: SourceProductName=HCU Relative Block Library
  Switch : Switch  Criteria=u2 > Threshold
  VPMM_RlyOpenCheck_flg : Outport  VectorParamsAs1DForOutWhenUnconnected=off
  VPMM_HVUnitSelfChkCompleted4PU_flg : Outport  Port=2  VectorParamsAs1DForOutWhenUnconnected=off
  VPMM_HVUnitSelfChkCompleted4Chrg_flg : Outport  Port=3  VectorParamsAs1DForOutWhenUnconnected=off
  VPMM_HVFailureChkPass_flg : Outport  Port=4
  wires:
  NOT5/1 -> SR_Latch1/1
  Equal/1 -> NOT5/1, Fault1/2
  SR_Latch3/1 -> AND2/4
  [task_time_s] -> Fault3/1
  NOT4/1 -> Fault3/2
  Constant23/1 -> Fault3/3
  Switch/1 -> SR_Latch3/1, NOT4/1
  Fault3/1 -> SR_Latch3/2
  SR_Latch2/1 -> AND2/3
  Fault2/1 -> SR_Latch2/2
  [VPMM_PDUNoFail_flg] -> NOT3/1, SR_Latch2/1
  Constant22/1 -> Fault2/3
  NOT3/1 -> Fault2/2
  [task_time_s] -> Fault2/1
  [task_time_s] -> Fault1/1
  Constant21/1 -> Fault1/3
  Fault1/1 -> SR_Latch1/2
  SR_Latch1/1 -> AND2/2
  Fault/1 -> SR_Latch/2
  Constant20/1 -> Fault/3
  [task_time_s] -> Fault/1
  task_time_s/1 -> [task_time_s]
  SR_Latch/1 -> AND2/1
  NOT1/1 -> SR_Latch/1
  Constant19/1 -> Switch/1
  Constant18/1 -> Switch/2
  [VPMM_MCUNoFail_flg] -> Switch/3
  AND2/1 -> VPMM_HVFailureChkPass_flg/1  "VPMM_HVFailureChkPass_flg"
  Constant/1 -> Equal/2
  VINP_HVPwrOffReq_enum/1 -> Equal/1
  VPMM_HVILFail_flg/1 -> NOT1/1, Fault/2
  Relational Operator11/1 -> Logical Operator/9
  Relational Operator14/1 -> Logical Operator/10
  Relational Operator15/1 -> Logical Operator/11
  Relational Operator16/1 -> Logical Operator/12
  Constant16/1 -> Relational Operator16/2
  Constant15/1 -> Relational Operator15/2
  Constant14/1 -> Relational Operator14/2
  Constant11/1 -> Relational Operator11/2
  VINP_MCUHVLoopSts_enum/1 -> Relational Operator16/1
  VINP_B2VDCChgN1RlySta_enum/1 -> Relational Operator15/1
  VINP_B2VDCChgP1RlySta_enum/1 -> Relational Operator14/1
  VINP_B2VMainNegRlySta_enum/1 -> Relational Operator11/1
  NOT/1 -> AND/1, AND1/1
  Constant13/1 -> Relational Operator13/2
  VINP_B2VFaultCode_enum/1 -> Relational Operator13/1
  VINP_B2VHVILFault_flg/1 -> NOT/1
  AND1/1 -> VPMM_HVUnitSelfChkCompleted4Chrg_flg/1  "VPMM_HVUnitSelfChkCompleted4Chrg_flg"
  Relational Operator12/1 -> AND/5
  Relational Operator10/1 -> AND1/3, AND/3, [VPMM_PDUNoFail_flg]
  Relational Operator7/1 -> AND/4, [VPMM_MCUNoFail_flg]
  Relational Operator13/1 -> AND/2, AND1/2
  Constant12/1 -> Relational Operator12/2
  VINP_MCUFailCode_enum/1 -> Relational Operator12/1
  Constant9/1 -> Relational Operator7/2
  VINP_MCUFailGrade_enum/1 -> Relational Operator7/1
  Constant4/1 -> Relational Operator2/2
  Constant6/1 -> Relational Operator4/2
  Constant7/1 -> Relational Operator5/2
  Constant5/1 -> Relational Operator3/2
  VSCP_PDUEHPSRlySta_enum/1 -> Relational Operator3/1
  Constant10/1 -> Relational Operator8/2
  VSCP_PDUDCDCRlySta_enum/1 -> Relational Operator2/1
  VINP_ACPrechrgRlySts_enum/1 -> Relational Operator5/1
  VSCP_PDUEACRlySta_enum/1 -> Relational Operator4/1
  VINP_MCUPrechrgRlySts_enum/1 -> Relational Operator8/1
  Relational Operator8/1 -> Logical Operator/7
  Relational Operator5/1 -> Logical Operator/6
  Relational Operator4/1 -> Logical Operator/5
  Relational Operator3/1 -> Logical Operator/4
  Relational Operator2/1 -> Logical Operator/3
  Logical Operator/1 -> VPMM_RlyOpenCheck_flg/1  "VPMM_RlyOpenCheck_flg"
  Constant1/1 -> Relational Operator1/2
  VINP_BMSHVSts_enum/1 -> Relational Operator1/1
  Relational Operator1/1 -> Logical Operator/2
  Relational Operator9/1 -> Logical Operator/1
  VINP_PDUMCUPosRlySta_enum/1 -> Relational Operator9/1
  Constant2/1 -> Relational Operator9/2
  Constant3/1 -> Relational Operator10/2
  VINP_PEUSelfChkSts_enum/1 -> Relational Operator10/1
  Constant8/1 -> Relational Operator6/2
  VINP_PDUACRlySta_enum/1 -> Relational Operator6/1
  Relational Operator6/1 -> Logical Operator/8
  AND/1 -> VPMM_HVUnitSelfChkCompleted4PU_flg/1  "VPMM_HVUnitSelfChkCompleted4PU_flg"

== system pmm/PMM/PowerModeManagement/PMM State Change Configuration/PMM AfterRun to Initialize State ==
  note: [(VPSA_Keystatus_enum == ENUM_KEYSTATUS_ON)]
  VPSA_Keystatus_enum : Inport
  Constant2 : Constant  Value=ENUM_KEYSTATUS_ON
  Equal : RelationalOperator  Operator===  OutDataTypeStr=boolean  RndMeth=Simplest
  VPMM_AfterRun2Initialize_flg : Outport
  wires:
  [VPSA_Keystatus_enum] -> Equal/1
  VPSA_Keystatus_enum/1 -> [VPSA_Keystatus_enum]
  Constant2/1 -> Equal/2
  Equal/1 -> VPMM_AfterRun2Initialize_flg/1  "VPMM_AfterRun2Initialize_flg"

== system pmm/PMM/PowerModeManagement/PMM State Change Configuration/PMM Boot to Initialize State ==
  note: ((VPSA_Keystatus_enum == ENUM_KEYSTATUS_ON) || (VPSA_Keystatus_enum == ENUM_KEYSTATUS_START) || (VINP_ChargeWakeup_flg)) &&...
      | VPMM_ChrgwakeDebon_cnt > KPMM_ChrgwakeDebon_cnt
      | ]
  VPSA_Keystatus_enum : Inport
  VINP_ChargeWakeup_flg : Inport  Port=2
  Constant1 : Constant  Value=ENUM_KEYSTATUS_START
  Constant45 : Constant  Value=ENUM_KEYSTATUS_ON
  OR : Logic  Operator=OR  Inputs=3  AllPortsSameDT=off  OutDataTypeStr=boolean
  Relational Operator : RelationalOperator  Operator===  OutDataTypeStr=boolean  RndMeth=Simplest
  Relational Operator1 : RelationalOperator  Operator===  OutDataTypeStr=boolean  RndMeth=Simplest
  VPMM_Boot2Initialize_flg : Outport
  wires:
  Constant1/1 -> Relational Operator1/2
  Relational Operator1/1 -> OR/2
  [VPSA_Keystatus_enum] -> Relational Operator/1
  [VPSA_Keystatus_enum] -> Relational Operator1/1
  Constant45/1 -> Relational Operator/2
  OR/1 -> VPMM_Boot2Initialize_flg/1  "VPMM_Boot2Initialize_flg"
  Relational Operator/1 -> OR/1
  [VINP_ChargeWakeup_flg] -> OR/3
  VPSA_Keystatus_enum/1 -> [VPSA_Keystatus_enum]
  VINP_ChargeWakeup_flg/1 -> [VINP_ChargeWakeup_flg]

== system pmm/PMM/PowerModeManagement/PMM State Change Configuration/PMM Charge to PowerDown State ==
  note: [VPMM_ChrgIntoPwrdown_flg ||
      | VPMM_LostCom_flg ||
      | VPMM_RCIncorrect_flg ||...
      | VDMM_WireFailure_flg]
  VPMM_LostCom_flg : Inport
  VPMM_RCIncorrect_flg : Inport  Port=2
  VDMM_DTCVCUPowerVolHigh_flg : Inport  Port=3
  VDMM_DTCVCUPowerVolLow_flg : Inport  Port=4
  VDMM_DTCHVILWireFailure_flg : Inport  Port=5
  VDMM_WireFailure_flg : Inport  Port=6
  OR : Logic  Operator=OR  Inputs=6  AllPortsSameDT=off  OutDataTypeStr=boolean
  VPMM_Charge2PowerDown_flg : Outport
  wires:
  VPMM_RCIncorrect_flg/1 -> [VPMM_RCIncorrect_flg]
  VPMM_LostCom_flg/1 -> [VPMM_LostCom_flg]
  [VPMM_LostCom_flg] -> OR/1
  OR/1 -> VPMM_Charge2PowerDown_flg/1  "VPMM_Charge2PowerDown_flg"
  [VPMM_RCIncorrect_flg] -> OR/2
  VDMM_DTCVCUPowerVolHigh_flg/1 -> [VDMM_DTCVCUPowerVolHigh_flg]
  VDMM_DTCVCUPowerVolLow_flg/1 -> [VDMM_DTCVCUPowerVolLow_flg]
  VDMM_DTCHVILWireFailure_flg/1 -> [VDMM_DTCHVILWireFailure_flg]
  [VDMM_DTCVCUPowerVolHigh_flg] -> OR/3
  [VDMM_DTCVCUPowerVolLow_flg] -> OR/4
  [VDMM_DTCHVILWireFailure_flg] -> OR/5
  VDMM_WireFailure_flg/1 -> [VDMM_WireFailure_flg]
  [VDMM_WireFailure_flg] -> OR/6

== system pmm/PMM/PowerModeManagement/PMM State Change Configuration/PMM Drive to PowerDown State ==
  note: [VPSA_Keystatus_enum == ENUM_KEYSTATUS_OFF ||...
      | VPSA_EmergencyShutDown_flg ||...
      | VPMM_HVILEmergencyStop_flg ||...
      | VPMM_LostCom_flg ||...
      | VPMM_RCIncorrect_flg ||...
      | VDMM_WireFailure_flg ||...
      | VPMM_LVChrgFinished_flg||...
      | (VPMM_SysPowerMode_enum ==ENUM_PMMMODE_LVBATCHRG && VINP_B2VSOC_pct < KPMM_LVChrgEnHVSOC_pct)]
  VPSA_Keystatus_enum : Inport
  VPSA_EmergencyShutDown_flg : Inport  Port=2
  VPMM_HVILEmergencyStop_flg : Inport  Port=3
  VPMM_LostCom_flg : Inport  Port=4
  VPMM_RCIncorrect_flg : Inport  Port=5
  VDMM_DTCVCUPowerVolHigh_flg : Inport  Port=6
  VDMM_DTCVCUPowerVolLow_flg : Inport  Port=7
  VDMM_DTCHVILWireFailure_flg : Inport  Port=8
  VPMM_HVRlyNoFeedBack_flg : Inport  Port=9
  VDMM_WireFailure_flg : Inport  Port=10
  VINP_B2VSOC_pct : Inport  Port=11
  VPMM_SysPowerMode_enum : Inport  Port=12
  VPMM_LVChrgFinished_flg : Inport  Port=13
  VINP_ParkBrakeSW_flg : Inport  Port=14
  VSCP_LVchrgSvrMode_flg : Inport  Port=15
  VPMM_LongIdle_flg : Inport  Port=16
  AND : Logic  AllPortsSameDT=off  OutDataTypeStr=boolean
  Constant1 : Constant  Value=ENUM_PMMMODE_LVBATCHRG
  Constant2 : Constant  Value=ENUM_KEYSTATUS_OFF
  Equal : RelationalOperator  Operator===  OutDataTypeStr=boolean  RndMeth=Simplest
  Equal1 : RelationalOperator  Operator===  OutDataTypeStr=boolean  RndMeth=Simplest
  NOT : Logic  Operator=NOT  AllPortsSameDT=off  OutDataTypeStr=boolean
  NOT1 : Logic  Operator=NOT  AllPortsSameDT=off  OutDataTypeStr=boolean
  OR : Logic  Operator=OR  Inputs=13  AllPortsSameDT=off  OutDataTypeStr=boolean
  OR1 : Logic  Operator=OR  Inputs=3  AllPortsSameDT=off  OutDataTypeStr=boolean
  Relay : Relay  OnSwitchValue=KPMM_LVChrgEnHVSOC_pct  OffSwitchValue=KPMM_LVChrgDisHVSOC_pct  OnOutputValue=TRUE  OffOutputValue=FALSE  OutDataTypeStr=boolean
  VPMM_Drive2PowerDown_flg : Outport
  wires:
  [VPMM_HVILEmergencyStop_flg] -> OR/3
  VPMM_HVILEmergencyStop_flg/1 -> [VPMM_HVILEmergencyStop_flg]
  [VPMM_LostCom_flg] -> OR/4
  [VPSA_EmergencyShutDown_flg] -> OR/2
  [VPMM_RCIncorrect_flg] -> OR/5
  Constant2/1 -> Equal/2
  [VPSA_Keystatus_enum] -> Equal/1
  VPSA_EmergencyShutDown_flg/1 -> [VPSA_EmergencyShutDown_flg]
  VPMM_LostCom_flg/1 -> [VPMM_LostCom_flg]
  VPSA_Keystatus_enum/1 -> [VPSA_Keystatus_enum]
  VPMM_RCIncorrect_flg/1 -> [VPMM_RCIncorrect_flg]
  Equal/1 -> OR/1
  OR/1 -> VPMM_Drive2PowerDown_flg/1  "VPMM_Drive2PowerDown_flg"
  VDMM_DTCHVILWireFailure_flg/1 -> [VDMM_DTCHVILWireFailure_flg]
  VDMM_DTCVCUPowerVolLow_flg/1 -> [VDMM_DTCVCUPowerVolLow_flg]
  VDMM_DTCVCUPowerVolHigh_flg/1 -> [VDMM_DTCVCUPowerVolHigh_flg]
  [VDMM_DTCVCUPowerVolHigh_flg] -> OR/6
  [VDMM_DTCVCUPowerVolLow_flg] -> OR/7
  [VDMM_DTCHVILWireFailure_flg] -> OR/8
  VPMM_HVRlyNoFeedBack_flg/1 -> [VPMM_HVRlyNoFeedBack_flg]
  [VPMM_HVRlyNoFeedBack_flg] -> OR/9
  VDMM_WireFailure_flg/1 -> [VDMM_WireFailure_flg]
  [VDMM_WireFailure_flg] -> OR/10
  VINP_B2VSOC_pct/1 -> [VINP_B2VSOC_pct]
  VPMM_SysPowerMode_enum/1 -> [VPMM_SysPowerMode_enum]
  [VPMM_SysPowerMode_enum] -> Equal1/1
  Constant1/1 -> Equal1/2
  [VINP_B2VSOC_pct] -> Relay/1
  Equal1/1 -> AND/1
  VPMM_LVChrgFinished_flg/1 -> [VPMM_LVChrgFinished_flg]
  [VPMM_LVChrgFinished_flg] -> OR/11
  OR1/1 -> AND/2
  VINP_ParkBrakeSW_flg/1 -> [VINP_ParkBrakeSW_flg]
  NOT/1 -> OR1/2
  [VINP_ParkBrakeSW_flg] -> NOT/1
  [VSCP_LVchrgSvrMode_flg] -> OR1/3
  VSCP_LVchrgSvrMode_flg/1 -> [VSCP_LVchrgSvrMode_flg]
  Relay/1 -> NOT1/1
  NOT1/1 -> OR1/1
  VPMM_LongIdle_flg/1 -> [VPMM_LongIdle_flg]
  AND/1 -> OR/13
  [VPMM_LongIdle_flg] -> OR/12

== system pmm/PMM/PowerModeManagement/PMM State Change Configuration/PMM Initialize to Charge State ==
  note: [(VINP_ChargeWakeup_flg) && (VPMM_HVSelfChkCompleted4Chrg_flg) && ...
      |  (VINP_DCChrgConnectSts_enum == ENUM_PLUGINSTS_PLUGIN) && ...
      |  (VPSA_Keystatus_enum == ENUM_KEYSTATUS_OFF) && ...
      |  (!VPMM_HVILEmergencyStop_flg)&&...
      |  (!VDMM_ProhibitCharge_flg)]
  VINP_ChargeWakeup_flg : Inport
  VINP_DCChrgConnectSts_enum : Inport  Port=2
  VPSA_Keystatus_enum : Inport  Port=3
  VPMM_HVILEmergencyStop_flg : Inport  Port=4
  VDMM_ProhibitCharge_flg : Inport  Port=5
  AND : Logic  Inputs=5  AllPortsSameDT=off  OutDataTypeStr=boolean
  Constant2 : Constant  Value=ENUM_PLUGINSTS_PLUGIN
  Constant3 : Constant  Value=ENUM_KEYSTATUS_OFF
  NOT : Logic  Operator=NOT  AllPortsSameDT=off  OutDataTypeStr=boolean
  NOT1 : Logic  Operator=NOT  AllPortsSameDT=off  OutDataTypeStr=boolean
  Relational Operator : RelationalOperator  Operator===  OutDataTypeStr=boolean  RndMeth=Simplest
  Relational Operator1 : RelationalOperator  Operator===  OutDataTypeStr=boolean  RndMeth=Simplest
  VPMM_Initialize2Charge_flg : Outport
  wires:
  VINP_DCChrgConnectSts_enum/1 -> [VINP_DCChrgConnectSts_enum]
  VPSA_Keystatus_enum/1 -> [VPSA_Keystatus_enum]
  VINP_ChargeWakeup_flg/1 -> [VINP_ChargeWakeup_flg]
  Constant3/1 -> Relational Operator/2
  [VPMM_HVILEmergencyStop_flg] -> NOT/1
  VPMM_HVILEmergencyStop_flg/1 -> [VPMM_HVILEmergencyStop_flg]
  [VINP_DCChrgConnectSts_enum] -> Relational Operator1/1
  [VINP_ChargeWakeup_flg] -> AND/1
  [VPSA_Keystatus_enum] -> Relational Operator/1
  Constant2/1 -> Relational Operator1/2
  AND/1 -> VPMM_Initialize2Charge_flg/1  "VPMM_Initialize2Charge_flg"
  Relational Operator1/1 -> AND/2
  Relational Operator/1 -> AND/3
  NOT/1 -> AND/4
  VDMM_ProhibitCharge_flg/1 -> [VDMM_ProhibitCharge_flg]
  [VDMM_ProhibitCharge_flg] -> NOT1/1
  NOT1/1 -> AND/5

== system pmm/PMM/PowerModeManagement/PMM State Change Configuration/PMM Initialize to Idle State ==
  note: [(VPSA_Keystatus_enum == ENUM_KEYSTATUS_OFF && !VINP_ChargeWakeup_flg) ||...
      | (VPMM_SysInitialTO_flg )
      | ||...
      | (VPMM_DCDCVolLowTO_flg &&
      | (VSCP_LVchrgSvrMode_flg || !VINP_ParkBrakeSW_flg || VINP_B2VSOC_pct < KPMM_LVChrgDisHVSOC_pct))]
  VPSA_Keystatus_enum : Inport
  VINP_ChargeWakeup_flg : Inport  Port=2
  VPMM_LVChrgPreActFinished_flg : Inport  Port=3
  VSCP_LVchrgSvrMode_flg : Inport  Port=4
  VINP_ParkBrakeSW_flg : Inport  Port=5
  VINP_B2VSOC_pct : Inport  Port=6
  AND : Logic  AllPortsSameDT=off  OutDataTypeStr=boolean
  AND1 : Logic  Operator=OR  AllPortsSameDT=off  OutDataTypeStr=boolean
  AND2 : Logic  AllPortsSameDT=off  OutDataTypeStr=boolean
  Constant45 : Constant  Value=ENUM_KEYSTATUS_OFF
  NOT : Logic  Operator=NOT  AllPortsSameDT=off  OutDataTypeStr=boolean
  NOT1 : Logic  Operator=NOT  AllPortsSameDT=off  OutDataTypeStr=boolean
  NOT2 : Logic  Operator=NOT  AllPortsSameDT=off  OutDataTypeStr=boolean
  OR : Logic  Operator=OR  Inputs=3  AllPortsSameDT=off  OutDataTypeStr=boolean
  Relational Operator : RelationalOperator  Operator===  OutDataTypeStr=boolean  RndMeth=Simplest
  Relay : Relay  OnSwitchValue=KPMM_LVChrgEnHVSOC_pct  OffSwitchValue=KPMM_LVChrgDisHVSOC_pct  OnOutputValue=TRUE  OffOutputValue=FALSE  OutDataTypeStr=boolean
  VPMM_Initialize2Idle_flg : Outport
  VPMM_LVChrgIinit2Idle_flg : Outport  Port=2
  wires:
  AND/1 -> AND1/1
  [VPSA_Keystatus_enum] -> Relational Operator/1
  Constant45/1 -> Relational Operator/2
  Relational Operator/1 -> AND/1
  AND1/1 -> VPMM_Initialize2Idle_flg/1  "VPMM_Initialize2Idle_flg"
  VPSA_Keystatus_enum/1 -> [VPSA_Keystatus_enum]
  VPMM_LVChrgPreActFinished_flg/1 -> [VPMM_LVChrgPreActFinished_flg]
  VINP_ChargeWakeup_flg/1 -> [VINP_ChargeWakeup_flg]
  NOT/1 -> AND/2
  [VINP_ChargeWakeup_flg] -> NOT/1
  VSCP_LVchrgSvrMode_flg/1 -> [VSCP_LVchrgSvrMode_flg]
  [VPMM_LVChrgPreActFinished_flg] -> AND2/1
  AND2/1 -> VPMM_LVChrgIinit2Idle_flg/1, AND1/2  "VPMM_LVChrgIinit2Idle_flg"
  [VSCP_LVchrgSvrMode_flg] -> OR/1
  [VINP_ParkBrakeSW_flg] -> NOT1/1
  NOT1/1 -> OR/2
  [VINP_B2VSOC_pct] -> Relay/1
  OR/1 -> AND2/2
  VINP_ParkBrakeSW_flg/1 -> [VINP_ParkBrakeSW_flg]
  VINP_B2VSOC_pct/1 -> [VINP_B2VSOC_pct]
  Relay/1 -> NOT2/1
  NOT2/1 -> OR/3
